simulink model "sistem_oscilant"  (R2023b)
settings: Solver=ode45  StartTime=0.0  StopTime=150  MaxStep=1e-3  RelTol=1e-3
values from neighbouring files (symbols this model uses):
  b = 0.2    [sns_proiect_Ceoca_Ovidiu.m]
  den = [T 1]    [sns_proiect_Ceoca_Ovidiu.m]
  h1 = T/10    (= 0.2)    [sns_proiect_Ceoca_Ovidiu.m]
  Kp = 0.45*Ku    (= 0.450881601519)    [sns_proiect_Ceoca_Ovidiu.m]
  num = [1]    [sns_proiect_Ceoca_Ovidiu.m]
  sat_value = 2    [sns_proiect_Ceoca_Ovidiu.m]
  Ti = 0.8*Tosc    (= 8)    [sns_proiect_Ceoca_Ovidiu.m]
  Tt1 = 0.5    [sns_proiect_Ceoca_Ovidiu.m]
settings Model: Creator=ovidiuceoca  LastModifiedBy=ovidiuceoca

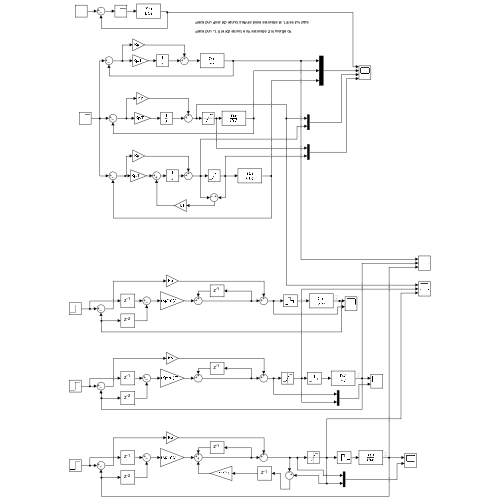
[thumbnail: Simulink's stored preview of the top-level diagram]
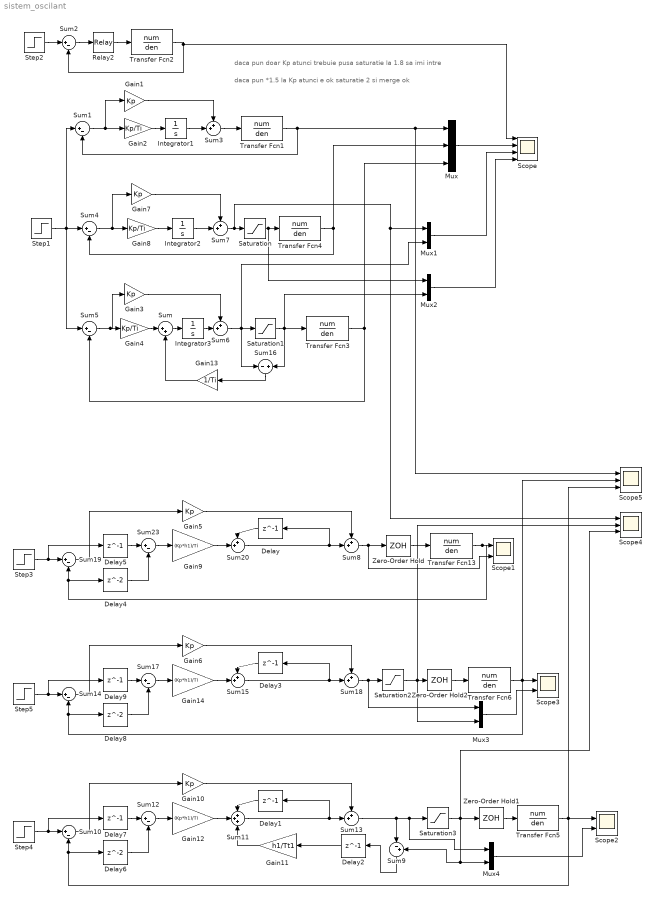
== system sistem_oscilant ==
  note: daca pun *1.5 la Kp atunci e ok saturatie 2 si merge ok
  note: daca pun doar Kp atunci trebuie pusa saturatie la 1.8 sa imi intre
  Delay{,1..3,5,7,9} (7 alike) : Delay  DelayLength=1  SampleTime=h1
  Delay4 : Delay  SampleTime=h1
  Delay6 : Delay  SampleTime=h1
  Delay8 : Delay  SampleTime=h1
  Gain{1,3,5..7,10} (6 alike) : Gain  Gain=Kp
  Gain11 : Gain  Gain=h1/Tt1
  Gain12 : Gain  Gain=(Kp*h1)/Ti
  Gain13 : Gain  Gain=1/Ti
  Gain14 : Gain  Gain=(Kp*h1)/Ti
  Gain2 : Gain  Gain=Kp/Ti
  Gain4 : Gain  Gain=Kp/Ti
  Gain8 : Gain  Gain=Kp/Ti
  Gain9 : Gain  Gain=(Kp*h1)/Ti
  Integrator1 : Integrator
  Integrator2 : Integrator
  Integrator3 : Integrator
  Mux : Mux  Inputs=3
  Mux{1..4} (4 alike) : Mux  Inputs=2
  Relay2 : Relay  OnSwitchValue=0  OffSwitchValue=0  OnOutputValue=b  OffOutputValue=-b
  Saturation : Saturate  UpperLimit=sat_value  LowerLimit=0
  Saturation1 : Saturate  UpperLimit=sat_value  LowerLimit=0
  Saturation2 : Saturate  UpperLimit=sat_value  LowerLimit=-sat_value
  Saturation3 : Saturate  UpperLimit=sat_value  LowerLimit=-1.2
  Scope : Scope  NumInputPorts=4
  Scope1 : Scope  NumInputPorts=2
  Scope2 : Scope  NumInputPorts=2
  Scope3 : Scope  NumInputPorts=2
  Scope4 : Scope  NumInputPorts=3
  Scope5 : Scope  NumInputPorts=3
  Step{1,3..5} (4 alike) : Step  Time=0  After=2  SampleTime=0
  Step2 : Step  Time=0  After=0.5  SampleTime=0
  Sum : Sum  Inputs=|++
  Sum{1..2,4..5,10,12,14,17,19,23} (10 alike) : Sum  Inputs=|+-
  Sum11 : Sum  Inputs=+++
  Sum{3,6..8,13,15,18,20} (8 alike) : Sum  Inputs=++|
  Sum16 : Sum  Inputs=-|+
  Sum9 : Sum  Inputs=|-+
  Transfer Fcn{1..6,13} (7 alike) : TransferFcn  Numerator=num  Denominator=den
  Zero-Order Hold : ZeroOrderHold  SampleTime=h1
  Zero-Order Hold1 : ZeroOrderHold  SampleTime=h1
  Zero-Order Hold2 : ZeroOrderHold  SampleTime=h1
  wires:
  Relay2/1 -> Transfer Fcn2/1
  Step2/1 -> Sum2/1
  Transfer Fcn2/1 -> Scope/1, Sum2/2
  Sum2/1 -> Relay2/1
  Integrator2/1 -> Sum7/2
  Gain7/1 -> Sum7/1
  Transfer Fcn4/1 -> Sum4/2, Mux/2
  Sum4/1 -> Gain8/1, Gain7/1
  Gain8/1 -> Integrator2/1
  Sum7/1 -> Scope4/1, Mux1/1, Saturation/1
  Saturation/1 -> Mux2/1, Transfer Fcn4/1
  Sum3/1 -> Transfer Fcn1/1
  Gain2/1 -> Integrator1/1
  Sum1/1 -> Gain1/1, Gain2/1
  Transfer Fcn1/1 -> Sum1/2, Scope5/1, Mux/1
  Gain1/1 -> Sum3/1
  Integrator1/1 -> Sum3/2
  Sum5/1 -> Gain3/1, Gain4/1
  Transfer Fcn3/1 -> Mux/3, Sum5/2
  Gain3/1 -> Sum6/1
  Integrator3/1 -> Sum6/2
  Gain13/1 -> Sum/2
  Sum6/1 -> Mux1/2, Sum16/1, Saturation1/1
  Saturation1/1 -> Mux2/2, Sum16/2, Transfer Fcn3/1
  Sum16/1 -> Gain13/1
  Sum/1 -> Integrator3/1
  Gain4/1 -> Sum/1
  Mux/1 -> Scope/2
  Mux1/1 -> Scope/3
  Mux2/1 -> Scope/4
  Sum19/1 -> Gain5/1
  Delay5/1 -> Sum23/1
  Sum20/1 -> Delay/1, Sum8/2
  Zero-Order Hold/1 -> Transfer Fcn13/1
  Gain5/1 -> Sum8/1
  Gain9/1 -> Sum20/2
  Delay4/1 -> Sum23/2
  Delay/1 -> Sum20/1
  Transfer Fcn13/1 -> Sum19/2, Delay4/1, Scope1/1
  Sum23/1 -> Gain9/1
  Step1/1 -> Sum1/1, Sum5/1, Sum4/1
  Sum8/1 -> Scope1/2, Zero-Order Hold/1
  Step3/1 -> Delay5/1, Sum19/1
  Gain10/1 -> Sum13/1
  Sum12/1 -> Gain12/1
  Mux4/1 -> Scope2/2
  Gain12/1 -> Sum11/2
  Delay7/1 -> Sum12/1
  Saturation3/1 -> Scope4/3, Zero-Order Hold1/1, Mux4/2, Sum9/2
  Delay6/1 -> Sum12/2
  Sum9/1 -> Delay2/1
  Delay1/1 -> Sum11/1
  Transfer Fcn5/1 -> Scope5/3, Sum10/2, Delay6/1, Scope2/1
  Delay2/1 -> Gain11/1
  Sum11/1 -> Delay1/1, Sum13/2
  Sum13/1 -> Sum9/1, Mux4/1, Saturation3/1
  Sum10/1 -> Gain10/1
  Step4/1 -> Delay7/1, Sum10/1
  Gain11/1 -> Sum11/3
  Zero-Order Hold1/1 -> Transfer Fcn5/1
  Sum18/1 -> Mux3/1, Saturation2/1
  Gain14/1 -> Sum15/2
  Gain6/1 -> Sum18/1
  Sum17/1 -> Gain14/1
  Delay3/1 -> Sum15/1
  Delay9/1 -> Sum17/1
  Delay8/1 -> Sum17/2
  Sum15/1 -> Delay3/1, Sum18/2
  Transfer Fcn6/1 -> Scope5/2, Sum14/2, Delay8/1, Scope3/1
  Sum14/1 -> Gain6/1
  Step5/1 -> Delay9/1, Sum14/1
  Zero-Order Hold2/1 -> Transfer Fcn6/1
  Saturation2/1 -> Scope4/2, Mux3/2, Zero-Order Hold2/1
  Mux3/1 -> Scope3/2
